simulink model "System"  (R2018a)
settings: Solver=FixedStepAuto  StartTime=0.0  StopTime=12000  FixedStep=0.01  RelTol=1e-3
libraries: simulink x1
settings Model: Creator=Kim  LastModifiedBy=kimnielsen

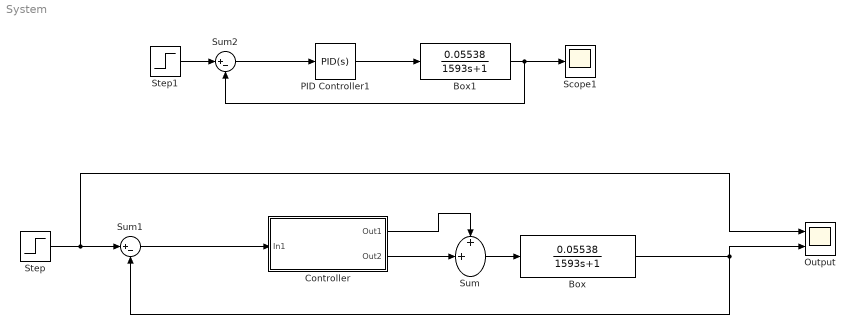
== system System ==
  Box : TransferFcn  Numerator=[0.05538]  Denominator=[1593 1]
  Box1 : TransferFcn  Numerator=[0.05538]  Denominator=[1593 1]
  Controller : Subsystem
  Output : Scope  NumInputPorts=2
  PID Controller1 : simulink/Continuous/PID Controller  Controller=PID  TimeDomain=Continuous-time  SampleTime=-1  IntegratorMethod=Forward Euler  FilterMethod=Forward Euler  Form=Parallel  UseFilter=on  ControllerParametersSource=internal  P=24.1527683964446  I=0.0303053974450705  D=-1397.28052246696  N=0.00237347247446869  InitialConditionSource=internal  InitialConditionForIntegrator=0  InitialConditionForFilter=0  ExternalReset=none  LimitOutput=off  UpperSaturationLimit=inf  LowerSaturationLimit=-inf  LinearizeAsGain=on  AntiWindupMode=none  Kb=1  TrackingMode=off  Kt=1  PParamMin=[]  PParamMax=[]  IParamMin=[]  IParamMax=[]  DParamMin=[]  DParamMax=[]  NParamMin=[]  NParamMax=[]  KbParamMin=[]  KbParamMax=[]  KtParamMin=[]  KtParamMax=[]  POutMin=[]  POutMax=[]  IOutMin=[]  IOutMax=[]  DOutMin=[]  DOutMax=[]  NOutMin=[]  NOutMax=[]  KbOutMin=[]  KbOutMax=[]  KtOutMin=[]  KtOutMax=[]  IntegratorOutMin=[]  IntegratorOutMax=[]  FilterOutMin=[]  FilterOutMax=[]  SumOutMin=[]  SumOutMax=[]  SumI1OutMin=[]  SumI1OutMax=[]  SumI2OutMin=[]  SumI2OutMax=[]  SumI3OutMin=[]  SumI3OutMax=[]  SumDOutMin=[]  SumDOutMax=[]  SaturationOutMin=[]  SaturationOutMax=[]  IntegratorContinuousStateAttributes=''  IntegratorStateMustResolveToSignalObject=off  IntegratorRTWStateStorageClass=Auto  FilterContinuousStateAttributes=''  FilterStateMustResolveToSignalObject=off  FilterRTWStateStorageClass=Auto  DifferentiatorICPrevScaledInput=0  DifferentiatorOutMin=[]  DifferentiatorOutMax=[]  FilterDiffOutCoefMin=[]  FilterDiffOutCoefMax=[]  SumDenOutMin=[]  SumDenOutMax=[]  SumNumOutMin=[]  SumNumOutMax=[]  ReciprocalOutMin=[]  ReciprocalOutMax=[]  DivideOutMin=[]  DivideOutMax=[]  TunerSelectOption=Transfer Function Based (PID Tuner App)
  Scope1 : Scope
  Step : Step  After=0.5  SampleTime=0
  Step1 : Step  After=0.5  SampleTime=0
  Sum : Sum  Inputs=++|
  Sum1 : Sum  Inputs=|+-
  Sum2 : Sum  Inputs=|+-
  wires:
  Sum/1 -> Box/1
  Step/1 -> Output/1, Sum1/1
  Box/1 -> Output/2, Sum1/2
  PID Controller1/1 -> Box1/1
  Box1/1 -> Scope1/1, Sum2/2
  Step1/1 -> Sum2/1
  Sum2/1 -> PID Controller1/1
  Sum1/1 -> Controller/1(In1)
  Controller/1(Out1) -> Sum/1
  Controller/2(Out2) -> Sum/2

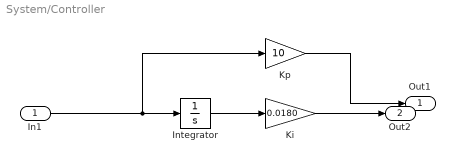
== system System/Controller ==
  In1 : Inport
  Integrator : Integrator
  Ki : Gain  Gain=0.0180
  Kp : Gain  Gain=10
  Out1 : Outport
  Out2 : Outport  Port=2
  wires:
  Ki/1 -> Out2/1
  Integrator/1 -> Ki/1
  Kp/1 -> Out1/1
  In1/1 -> Kp/1, Integrator/1
